simulink model "stace_space_model"  (R2020a)
settings: Solver=VariableStepAuto  StartTime=0.0  StopTime=1000  RelTol=1e-3
settings Model: Creator=啊包PC  LastModifiedBy=啊包PC

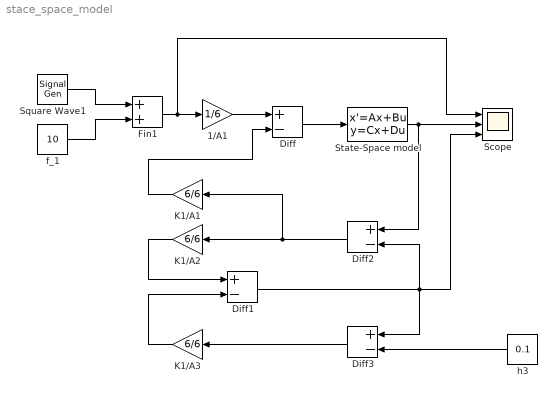
== system stace_space_model ==
  1/A1 : Gain  Gain=1/6
  Diff{,1..3} (4 alike) : Sum  Inputs=+-
  Fin1 : Sum
  K1/A1 : Gain  Gain=6/6
  K1/A2 : Gain  Gain=6/6
  K1/A3 : Gain  Gain=6/6
  Scope : Scope  NumInputPorts=3
  Square Wave1 : SignalGenerator  WaveForm=square  Amplitude=0.3*10  Frequency=1/60
  State-Space model : StateSpace  A=[1 -1; 1 -1/3]  B=[1/6 ; 1/75]  C=[1 0 ; 0 1]  D=[0 ; 0]  InitialCondition=0
  f_1 : Constant  Value=10
  h3 : Constant  Value=0.1
  wires:
  f_1/1 -> Fin1/2
  Square Wave1/1 -> Fin1/1
  Fin1/1 -> 1/A1/1, Scope/1
  State-Space model/1 -> Scope/2, Diff2/1
  h3/1 -> Diff3/2
  Diff3/1 -> K1/A3/1
  K1/A3/1 -> Diff1/2
  K1/A2/1 -> Diff1/1
  Diff1/1 -> Scope/3, Diff2/2, Diff3/1
  Diff2/1 -> K1/A1/1, K1/A2/1
  1/A1/1 -> Diff/1
  K1/A1/1 -> Diff/2
  Diff/1 -> State-Space model/1
